simulink model "tensegrity_structure"  (R2020b)
settings: Solver=ode45  StartTime=0.0  StopTime=60  MaxStep=0.001  RelTol=1e-3  AbsTol=1e-3  EnableMultiTasking=on
PreLoadFcn:
  | L=0.3;
  | K=100;
  | D=1;
model workspace (MAT data in the model file):
  L = 1
undefined symbols (not defined in the file): X, Y, Z
libraries: sm_lib x243, nesl_utility x19
(part 7 of 7)

== matlab function tensegrity_structure/onboard chip jump control/Actuators1-6/MATLAB Function ==
  data: time input; torque_17 output; jump input; idle_pre input; t0_pre input; torque_28 output; torque_39 output; torque_410 output; torque_511 output; torque_612 output; idle_new output; t0_new output; jump_pre input; jump_new output
function [torque_17,torque_28,torque_39,torque_410,torque_511,torque_612,idle_new,t0_new,jump_new] = jump(time,jump,idle_pre,t0_pre,jump_pre)
%%
t_now = time;
dt = 0.5;
max_torque = 25;
%%
if idle_pre == 1 % ready to jump
    if max(jump) == 1%jump
        idle_new = 0;
        t0_new = t_now;
        torque_17=0;torque_28=0;torque_39=0;torque_410=0;torque_511=0;torque_612=0;
        jump_new = jump;
    else % no jump
        idle_new = 1;
        t0_new = t_now;
        torque_17=0;torque_28=0;torque_39=0;torque_410=0;torque_511=0;torque_612=0;
        jump_new = zeros(6,1);
    end
else % idle_pre == 0;jump in progress
    if t_now <= t0_pre + dt % still have to compress
        idle_new = 0;
        t0_new = t0_pre;
        
        t_in = t_now - t0_pre;
        torque = max_torque*t_in/dt;
        
        torques = torque*jump_pre;  
        torque_17=torques(1);torque_28=torques(2);torque_39=torques(3);torque_410=torques(4);torque_511=torques(5);torque_612=torques(6);
        jump_new = jump_pre;
    else % compression completed
        idle_new = 1;
        t0_new = t_now;
        torque_17=0;torque_28=0;torque_39=0;torque_410=0;torque_511=0;torque_612=0;
        jump_new = zeros(6,1);
    end
        
end
    
    
    
    
end % end of function

== matlab function tensegrity_structure/onboard chip jump control/CPU/MATLAB Function ==
  data: z1 input; jump output; z2 input; z3 input; z4 input; z5 input; z6 input; z7 input; z8 input; z9 input; z10 input; z11 input; z12 input; delta_z_pre input; delta_z_new output
function  [jump, delta_z_new] = decide(z1,z2,z3,z4,z5,z6,z7,z8,z9,z10,z11,z12,delta_z_pre)
%%
threshold_z = 0.00002;
threshold_dz3 = 0.1;
isstatic = 0;
%%
dz17 = z1 - z7;
dz28 = z2 - z8;
dz39 = z3 - z9;
dz410 = z4 - z10;
dz511 = z5 - z11;
dz612 = z6 - z12;

% update
delta_z_new = [dz17;dz28;dz39;dz410;dz511;dz612];
% judge static
n_z = norm(delta_z_new - delta_z_pre);
if n_z < threshold_z % static
    isstatic = 1;
else
    isstatic = 0;
end
% output for mobile/static
if isstatic == 0 %mobile
    jump = zeros(6,1);
else %static
    % determine which two/one bar to jump
    zs = [z1;z2;z3;z4;z5;z6;z7;z8;z9;z10;z11;z12];
    zs_l2h = unique(zs);% low to high
    min_1 = find(zs==zs_l2h(1)); min_1 = mod(min_1-1,6)+1;
    min_2 = find(zs==zs_l2h(2)); min_2 = mod(min_2-1,6)+1;
    min_3 = find(zs==zs_l2h(3)); min_3 = mod(min_3-1,6)+1; % 1-6
    
    dzs_3 = [abs(delta_z_new(min_1));abs(delta_z_new(min_2));abs(delta_z_new(min_3))];
    if max(dzs_3) - min(dzs_3) > threshold_dz3 % two bars jump
        ids = [min_1;min_2;min_3];
        dontjump_dz = find(dzs_3 == min(dzs_3)); % most horizontal bar does't jump
        dontjump_id = ids(dontjump_dz);
        jump = zeros(6,1);
        jump(min_1) = 1;jump(min_2) = 1;jump(min_3) = 1;
        jump(dontjump_id)=0;
      
    else % one bar jump
        jump = zeros(6,1);
        jump(min_1) = 1;
    end
    delta_z_new = [dz17;dz28;dz39;dz410;dz511;dz612] + rand(6,1);% in case of static again
end

end %end of function
